simulink model "lane_keeping_control_system_by_DYC_block_diagram"  (R2018a)
settings: Solver=VariableStepAuto  StartTime=0.0  StopTime=8  RelTol=1e-3
undefined symbols (not defined in the file): C, Cf_M, Cr_M, D, dev, I_I, LCf_I, LCr_I, lf, lr, Ls, prop, V
settings Model: Creator=elbazam  LastModifiedBy=elbazam
settings DataIOCC: OutputOption=SpecifiedOutputTimes  OutputTimes=t

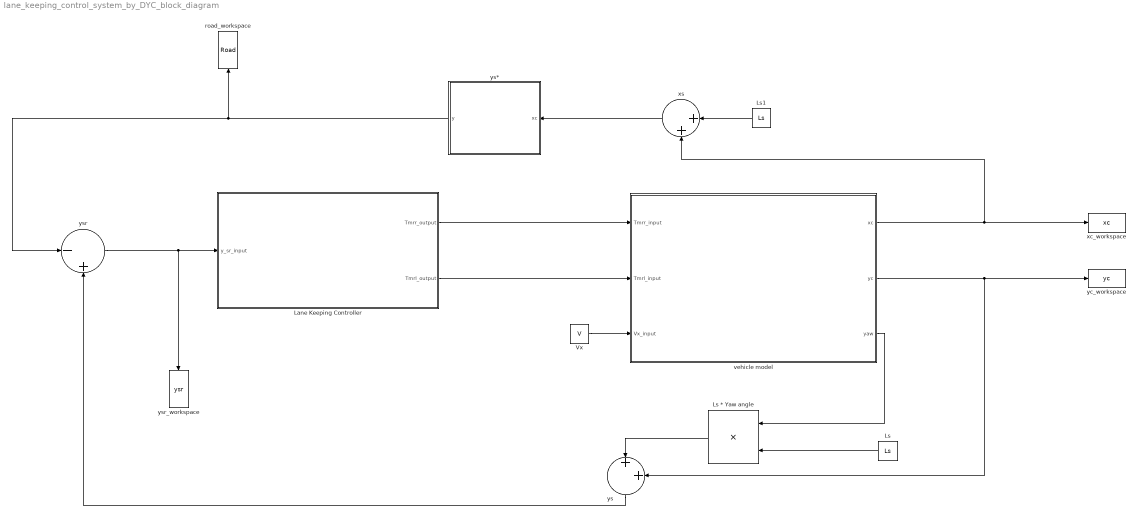
== system lane_keeping_control_system_by_DYC_block_diagram ==
  Lane Keeping Controller : Subsystem
  Ls : Constant  Value=Ls
  Ls * Yaw angle : Product
  Ls1 : Constant  Value=Ls
  Vx : Constant  Value=V
  road_workspace : ToWorkspace  VariableName=Road  SampleTime=-1
  vehicle model : Subsystem
  xc_workspace : ToWorkspace  VariableName=xc  SampleTime=-1
  xs : Sum  Inputs=|++
  yc_workspace : ToWorkspace  VariableName=yc  SampleTime=-1
  ys : Sum  Inputs=|++
  ys* : MATLAB Function  TreatAsAtomicUnit=on
  ysr : Sum  Inputs=|-+
  ysr_workspace : ToWorkspace  VariableName=ysr  SampleTime=-1
  wires:
  Lane Keeping Controller/2(Tmrl_output) -> vehicle model/2(Tmrl_input)
  Vx/1 -> vehicle model/3(Vx_input)
  vehicle model/1(xc) -> xs/2, xc_workspace/1
  vehicle model/2(yc) -> yc_workspace/1, ys/2
  vehicle model/3(yaw) -> Ls * Yaw angle/1
  Ls * Yaw angle/1 -> ys/1
  Ls/1 -> Ls * Yaw angle/2
  ysr/1 -> ysr_workspace/1, Lane Keeping Controller/1(y_sr_input)
  ys/1 -> ysr/2
  ys*/1(y) -> ysr/1, road_workspace/1
  Lane Keeping Controller/1(Tmrr_output) -> vehicle model/1(Tmrr_input)
  Ls1/1 -> xs/1
  xs/1 -> ys*/1(xc)

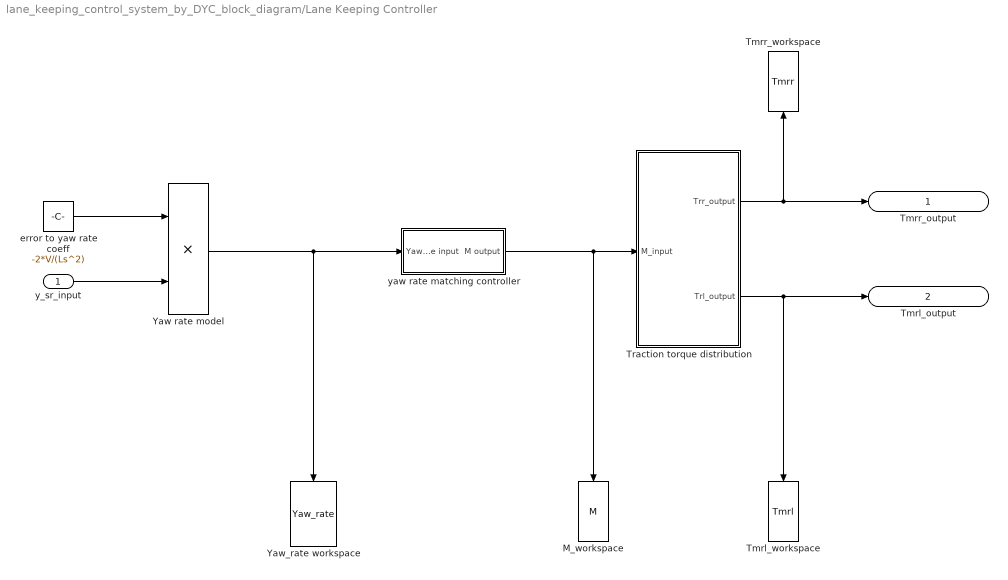
== system lane_keeping_control_system_by_DYC_block_diagram/Lane Keeping Controller ==
  y_sr_input : Inport
  M_workspace : ToWorkspace  VariableName=M  SampleTime=-1
  Tmrl_workspace : ToWorkspace  VariableName=Tmrl  SampleTime=-1
  Tmrr_workspace : ToWorkspace  VariableName=Tmrr  SampleTime=-1
  Traction torque distribution : Subsystem
  Yaw rate model : Product
  Yaw_rate workspace : ToWorkspace  VariableName=Yaw_rate  SampleTime=-1
  error to yaw rate coeff : Constant  Value=-2*V/(Ls^2)
  yaw rate matching controller : Subsystem
  Tmrr_output : Outport
  Tmrl_output : Outport  Port=2
  wires:
  y_sr_input/1 -> Yaw rate model/2
  Yaw rate model/1 -> yaw rate matching controller/1(Yaw rate input), Yaw_rate workspace/1
  yaw rate matching controller/1(M output) -> M_workspace/1, Traction torque distribution/1(M_input)
  Traction torque distribution/1(Trr_output) -> Tmrr_output/1, Tmrr_workspace/1
  Traction torque distribution/2(Trl_output) -> Tmrl_output/1, Tmrl_workspace/1
  error to yaw rate coeff/1 -> Yaw rate model/1

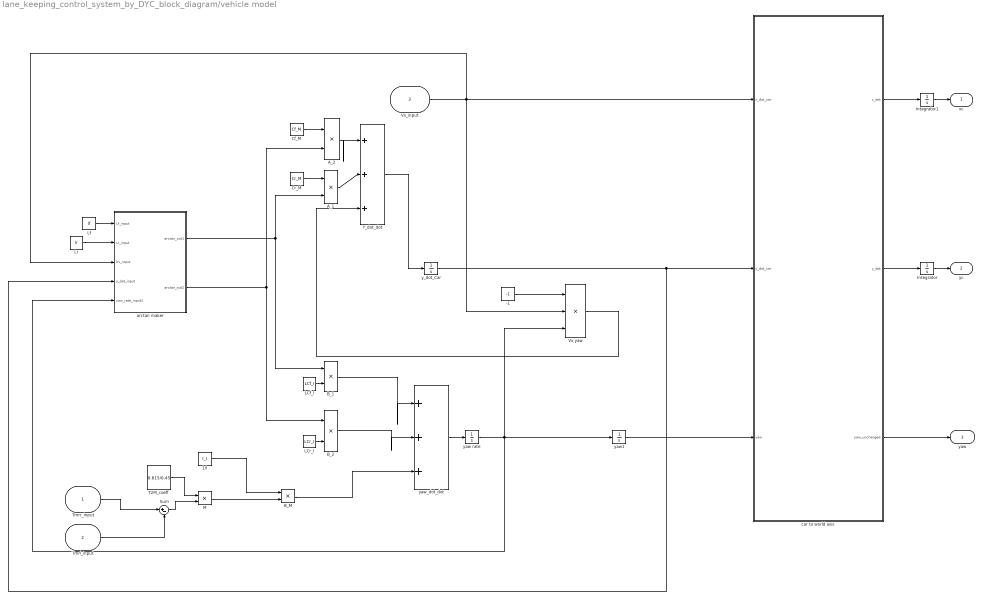
== system lane_keeping_control_system_by_DYC_block_diagram/vehicle model ==
  Tmrr_input : Inport
  Tmrl_input : Inport  Port=2
  Vx_input : Inport  Port=3
  -1 : Constant  Value=-1
  1/I : Constant  Value=I_I
  A_1 : Product
  A_2 : Product
  B_1 : Product
  B_2 : Product
  B_M : Product
  Cf_M : Constant  Value=Cf_M
  Cr_M : Constant  Value=Cr_M
  Integrator : Integrator
  Integrator1 : Integrator
  LCf_I : Constant  Value=LCf_I
  LCr_I : Constant  Value=LCr_I
  Lf : Constant  Value=lf
  Lr : Constant  Value=lr
  M : Product
  Sum : Sum  Inputs=|+-
  T2M_coeff : Constant  Value=0.815/0.45
  Vx yaw : Product  Inputs=3
  Y_dot_dot : Sum  Inputs=|+++
  arctan maker : Subsystem
  car to world axis : Subsystem
  y_dot_Car : Integrator
  yaw rate : Integrator
  yaw1 : Integrator
  yaw_dot_dot : Sum  Inputs=|+++
  xc : Outport
  yc : Outport  Port=2
  yaw : Outport  Port=3
  wires:
  Vx_input/1 -> Vx yaw/2, arctan maker/3(Vx_input), car to world axis/1(x_dot_car)
  Tmrl_input/1 -> Sum/2
  Tmrr_input/1 -> Sum/1
  T2M_coeff/1 -> M/1
  Sum/1 -> M/2
  car to world axis/3(yaw_unchanged) -> yaw/1
  Integrator/1 -> yc/1
  car to world axis/2(y_dot) -> Integrator/1
  car to world axis/1(x_dot) -> Integrator1/1
  Integrator1/1 -> xc/1
  M/1 -> B_M/2
  yaw_dot_dot/1 -> yaw rate/1
  yaw1/1 -> car to world axis/3(yaw)
  yaw rate/1 -> Vx yaw/3, yaw1/1, arctan maker/5(yaw_rate_input1)
  Y_dot_dot/1 -> y_dot_Car/1
  y_dot_Car/1 -> arctan maker/4(y_dot_input), car to world axis/2(y_dot_car)
  -1/1 -> Vx yaw/1
  Vx yaw/1 -> Y_dot_dot/3
  arctan maker/1(arctan_out1) -> A_1/2, B_1/1
  A_1/1 -> Y_dot_dot/2
  A_2/1 -> Y_dot_dot/1
  arctan maker/2(arctan_out2) -> A_2/2, B_2/1
  Cf_M/1 -> A_2/1
  Cr_M/1 -> A_1/1
  B_1/1 -> yaw_dot_dot/1
  B_2/1 -> yaw_dot_dot/2
  LCf_I/1 -> B_1/2
  LCr_I/1 -> B_2/2
  1/I/1 -> B_M/1
  B_M/1 -> yaw_dot_dot/3
  Lr/1 -> arctan maker/2(Lr_input)
  Lf/1 -> arctan maker/1(Lf_input)

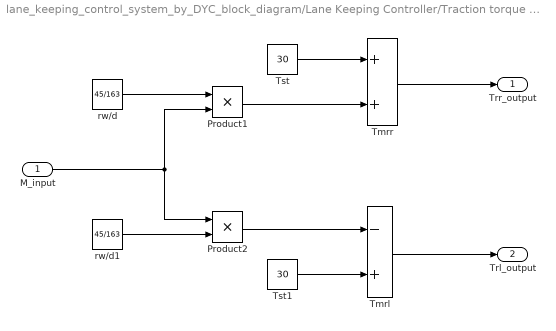
== system lane_keeping_control_system_by_DYC_block_diagram/Lane Keeping Controller/Traction torque distribution ==
  M_input : Inport
  Product1 : Product
  Product2 : Product
  Tmrl : Sum  Inputs=-+
  Tmrr : Sum
  Tst : Constant  Value=30
  Tst1 : Constant  Value=30
  rw/d : Constant  Value=45/163
  rw/d1 : Constant  Value=45/163
  Trr_output : Outport
  Trl_output : Outport  Port=2
  wires:
  Product2/1 -> Tmrl/1
  Product1/1 -> Tmrr/2
  rw/d/1 -> Product1/1
  M_input/1 -> Product2/1, Product1/2
  Tst1/1 -> Tmrl/2
  Tst/1 -> Tmrr/1
  rw/d1/1 -> Product2/2
  Tmrr/1 -> Trr_output/1
  Tmrl/1 -> Trl_output/1

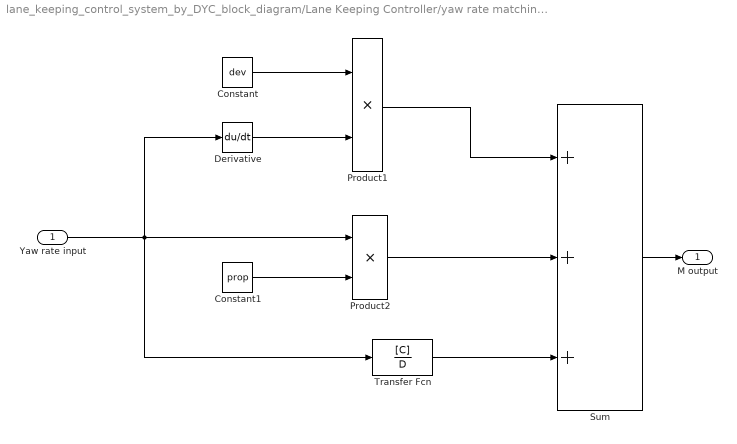
== system lane_keeping_control_system_by_DYC_block_diagram/Lane Keeping Controller/yaw rate matching controller ==
  Yaw rate input : Inport
  Constant : Constant  Value=dev
  Constant1 : Constant  Value=prop
  Derivative : Derivative
  Product1 : Product
  Product2 : Product
  Sum : Sum  Inputs=+++
  Transfer Fcn : TransferFcn  Numerator=[C]  Denominator=D
  M output : Outport
  wires:
  Yaw rate input/1 -> Transfer Fcn/1, Derivative/1, Product2/1
  Constant/1 -> Product1/1
  Derivative/1 -> Product1/2
  Constant1/1 -> Product2/2
  Sum/1 -> M output/1
  Product1/1 -> Sum/1
  Product2/1 -> Sum/2
  Transfer Fcn/1 -> Sum/3

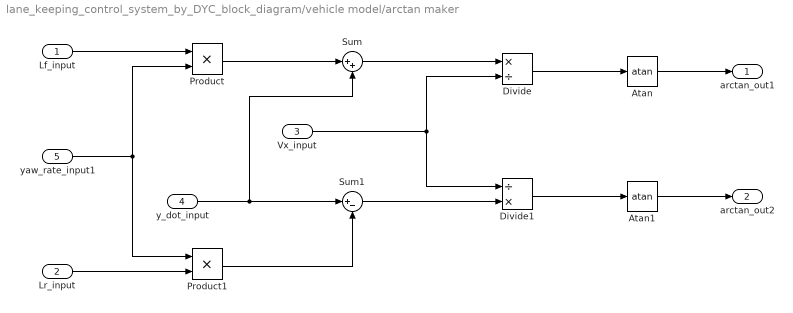
== system lane_keeping_control_system_by_DYC_block_diagram/vehicle model/arctan maker ==
  Lf_input : Inport
  Lr_input : Inport  Port=2
  Vx_input : Inport  Port=3
  y_dot_input : Inport  Port=4
  yaw_rate_input1 : Inport  Port=5
  Atan : Trigonometry  Operator=atan
  Atan1 : Trigonometry  Operator=atan
  Divide : Product  Inputs=*/
  Divide1 : Product  Inputs=/*
  Product : Product
  Product1 : Product
  Sum : Sum  Inputs=|++
  Sum1 : Sum  Inputs=|+-
  arctan_out1 : Outport
  arctan_out2 : Outport  Port=2
  wires:
  Lf_input/1 -> Product/1
  Lr_input/1 -> Product1/2
  Vx_input/1 -> Divide1/1, Divide/2
  y_dot_input/1 -> Sum/2, Sum1/1
  yaw_rate_input1/1 -> Product/2, Product1/1
  Product/1 -> Sum/1
  Product1/1 -> Sum1/2
  Divide/1 -> Atan/1
  Sum1/1 -> Divide1/2
  Sum/1 -> Divide/1
  Atan1/1 -> arctan_out2/1
  Atan/1 -> arctan_out1/1
  Divide1/1 -> Atan1/1

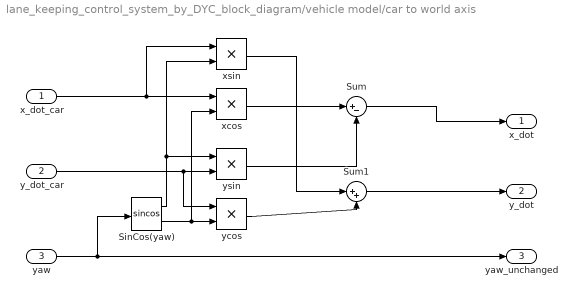
== system lane_keeping_control_system_by_DYC_block_diagram/vehicle model/car to world axis ==
  x_dot_car : Inport
  y_dot_car : Inport  Port=2
  yaw : Inport  Port=3
  SinCos(yaw) : Trigonometry  Operator=sincos
  Sum : Sum  Inputs=|+-
  Sum1 : Sum  Inputs=|++
  xcos : Product
  xsin : Product
  ycos : Product
  ysin : Product
  x_dot : Outport
  y_dot : Outport  Port=2
  yaw_unchanged : Outport  Port=3
  wires:
  x_dot_car/1 -> xsin/1, xcos/1
  yaw/1 -> SinCos(yaw)/1, yaw_unchanged/1
  y_dot_car/1 -> ycos/1, ysin/2
  SinCos(yaw)/1 -> ysin/1, xsin/2
  SinCos(yaw)/2 -> ycos/2, xcos/2
  xcos/1 -> Sum/1
  ysin/1 -> Sum/2
  Sum/1 -> x_dot/1
  ycos/1 -> Sum1/2
  xsin/1 -> Sum1/1
  Sum1/1 -> y_dot/1

== matlab function lane_keeping_control_system_by_DYC_block_diagram/ys* ==
  data: xc input; y output
function y = fcn(xc)

% if xc < 5
%     y = 0;
% else
%     y = sin(0.02*pi*xc)-sin(0.02*pi*5);
% end
if xc<25
    y = 0;
elseif xc > 25 && xc < 40
    y = (0.5/15)*(xc-25);
else
    y = 0.5;
end

end
